simulink model "single_phase_full_wave_rectifier"  (R2024b)
settings: Solver=ode3  StartTime=0.0  StopTime=4/50  FixedStep=10e-6  RelTol=1e-3
libraries: spsDiodeLib x8, spsVoltageMeasurementLib x3, spsSeriesRLCBranchLib x3, spsACVoltageSourceLib x2, sps_lib x1
settings Model: Creator=Abhijith_Kumble  LastModifiedBy=Abhijith_Kumble

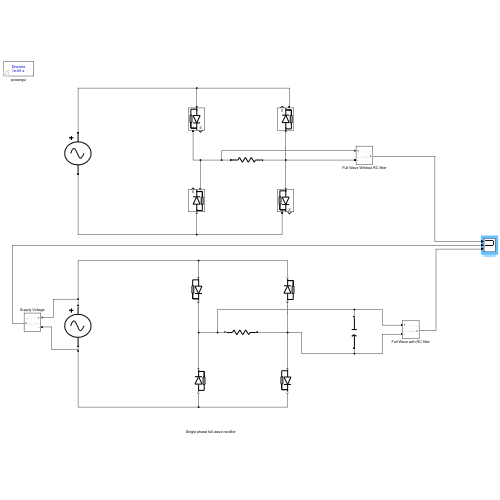
[thumbnail: Simulink's stored preview of the top-level diagram]
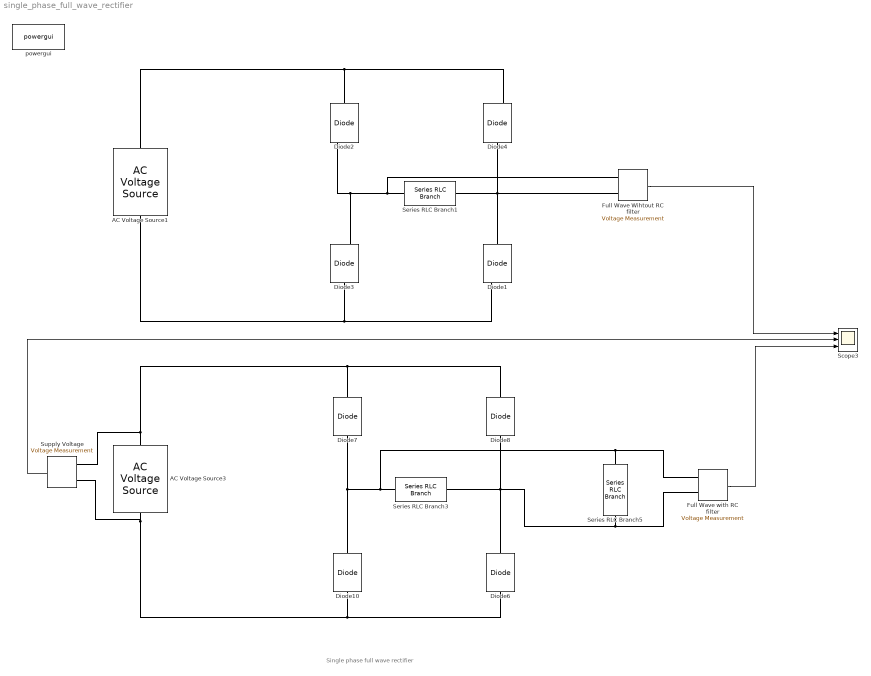
== system single_phase_full_wave_rectifier ==
  note: Single phase full wave rectifier
  AC Voltage Source1 : spsACVoltageSourceLib/AC Voltage Source  Amplitude=230  Phase=0  Frequency=50  SampleTime=0  Measurements=None  BusType=swing  Pref=10e3  Qref=0  Qmin=-inf  Qmax=+inf
  AC Voltage Source3 : spsACVoltageSourceLib/AC Voltage Source  Amplitude=230  Phase=0  Frequency=50  SampleTime=0  Measurements=None  BusType=swing  Pref=10e3  Qref=0  Qmin=-inf  Qmax=+inf
  Diode{1..4} (4 alike) : spsDiodeLib/Diode  Ron=0.001  Lon=0  Vf=0.8  IC=0  UseSnubber=0  Rs=500  Cs=250e-9  Measurements=on
  Diode{6..8,10} (4 alike) : spsDiodeLib/Diode  Ron=0.001  Lon=0  Vf=0.8  IC=0  UseSnubber=0  Rs=500  Cs=250e-9  Measurements=off
  Full Wave Wihtout RC filter : spsVoltageMeasurementLib/Voltage Measurement  PhasorSimulation=off  OutputType=Complex  PSBequivalent=0
  Full Wave with RC filter : spsVoltageMeasurementLib/Voltage Measurement  PhasorSimulation=off  OutputType=Complex  PSBequivalent=0
  Scope3 : Scope  NumInputPorts=3
  Series RLC Branch1 : spsSeriesRLCBranchLib/Series RLC Branch  LConnTagsString=__new0  RConnTagsString=__new0  BranchType=R  Resistance=1  Inductance=1e-3  SetiL0=off  InitialCurrent=0  Capacitance=1e-6  Setx0=off  InitialVoltage=0  Measurements=None
  Series RLC Branch3 : spsSeriesRLCBranchLib/Series RLC Branch  LConnTagsString=__new0  RConnTagsString=__new0  BranchType=R  Resistance=1000  Inductance=1e-3  SetiL0=off  InitialCurrent=0  Capacitance=1e-6  Setx0=off  InitialVoltage=0  Measurements=None
  Series RLC Branch5 : spsSeriesRLCBranchLib/Series RLC Branch  LConnTagsString=__new0  RConnTagsString=__new0  BranchType=C  Resistance=1  Inductance=1e-3  SetiL0=off  InitialCurrent=0  Capacitance=1e-3  Setx0=off  InitialVoltage=0  Measurements=None
  Supply Voltage : spsVoltageMeasurementLib/Voltage Measurement  PhasorSimulation=off  OutputType=Complex  PSBequivalent=0
  powergui : sps_lib/powergui  Priority=1  SimulationMode=Discrete  SampleTime=10e-6  frequency=50  Iterations=50  frequencyindice=50  Pbase=100e6  ErrMax=1e-4  UnitsV=kV  UnitsW=MW  buscounter=0  FunctionMessages=off  echomessages=off  EnableUseOfTLC=off  CurrentSourceSwitches=off  DisableSnubberDevices=off  DisableRonSwitches=off  DisableVfSwitches=off  DisplayEquations=off  AutomaticDiscreteSolvers=off  SolverType=Tustin/Backward Euler (TBE)  Interpol=off  ExternalGateDelay=off  methode=off  Ts=100  x0status=blocks  SPID=on  SwTol=0  HookPort=off  NonlinearTolerance=1e-4  nMaxIteration=100  ContinueOnMaxIteration=off  RestoreLinks=warning  ResistiveCurrentMeasurement=off  Frange=[0:2:500]  Ylog=off  Xlog=on  ShowGrid=off  save=off  variable=ZData  structure=0  ZoomFFT=off  StartTime=0.0  cycles=1  DisplayStyle=1  fundamental=60  FreqAxis=off  MaxFrequency=1000  frequencyindicesteady=1  RmsSteady=1  display=off
  wires:
  Full Wave Wihtout RC filter/1 -> Scope3/1
  Full Wave with RC filter/1 -> Scope3/3
  Supply Voltage/1 -> Scope3/2
  connections:
  AC Voltage Source1/RConn1 -- Diode4/RConn1 -- Diode2/LConn1
  AC Voltage Source1/LConn1 -- Diode1/RConn1 -- Diode3/LConn1
  Series RLC Branch1/LConn1 -- Full Wave Wihtout RC filter/LConn1 -- Diode2/RConn1 -- Diode3/RConn1
  Series RLC Branch1/RConn1 -- Diode4/LConn1 -- Diode1/LConn1 -- Full Wave Wihtout RC filter/LConn2
  AC Voltage Source3/RConn1 -- Supply Voltage/LConn1 -- Diode8/RConn1 -- Diode7/LConn1
  Series RLC Branch3/LConn1 -- Series RLC Branch5/LConn1 -- Full Wave with RC filter/LConn1 -- Diode7/RConn1 -- Diode10/RConn1
  Diode6/RConn1 -- Supply Voltage/LConn2 -- AC Voltage Source3/LConn1 -- Diode10/LConn1
  Full Wave with RC filter/LConn2 -- Diode6/LConn1 -- Diode8/LConn1 -- Series RLC Branch3/RConn1 -- Series RLC Branch5/RConn1
